simulink model "model"  (R2020b)
settings: Solver=VariableStepAuto  StartTime=0.0  StopTime=10.0  RelTol=1e-3
model workspace (MAT data in the model file):
  ki = Simulink.Parameter
  ki.Value = 10
  ki.DataType = 'auto'
  ki.Dimensions = [1 1]
  kp = Simulink.Parameter
  kp.Value = 10
  kp.DataType = 'auto'
  kp.Dimensions = [1 1]
  ts = Simulink.Parameter
  ts.Value = 1
  ts.DataType = 'auto'
  ts.Dimensions = [1 1]
settings Model: Creator=SAGAR  LastModifiedBy=SAGAR

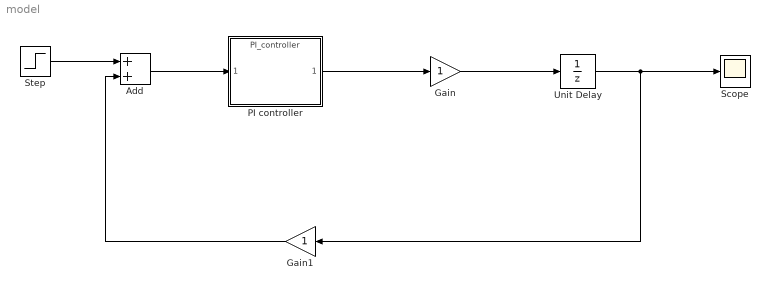
== system model ==
  Add : Sum
  Gain : Gain
  Gain1 : Gain
  PI controller : ModelReference  ModelNameDialog=PI_controller  SimulationMode=Normal  ModelReferenceVersion=1.2
  Scope : Scope
  Step : Step  SampleTime=0
  Unit Delay : UnitDelay  SampleTime=-1  HasFrameUpgradeWarning=on
  wires:
  Add/1 -> PI controller/1
  Step/1 -> Add/1
  PI controller/1 -> Gain/1
  Gain1/1 -> Add/2
  Gain/1 -> Unit Delay/1
  Unit Delay/1 -> Gain1/1, Scope/1
